simulink model "hopper_6dof_cascade_PID"  (R2025a)
settings: Solver=VariableStepAuto  StartTime=0.0  StopTime=36  RelTol=1e-3
undefined symbols (not defined in the file or in its folder): AVI, bp, ENGINE, IN, OUT, TANKS, tbl1, tbl2
libraries: slpidlib x13, dspindex x1, aerolibanim x1, SignalEditorBlockLib x1
(part 2 of 2)

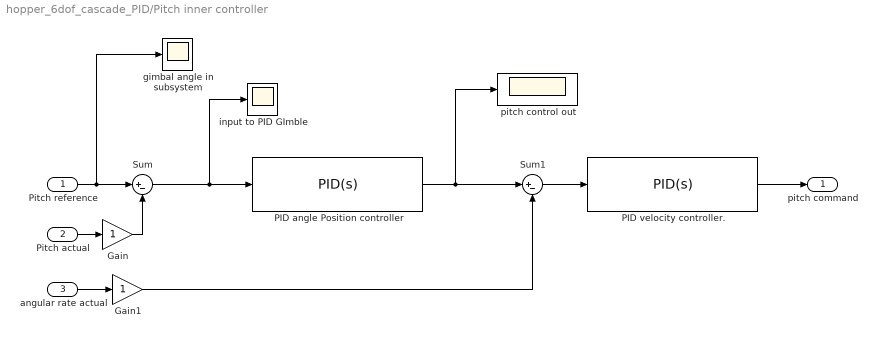
== system hopper_6dof_cascade_PID/Pitch inner controller ==
  Pitch reference : Inport
  Pitch actual : Inport  Port=2
  angular rate actual : Inport  Port=3
  Gain : Gain
  Gain1 : Gain
  PID angle Position controller : slpidlib/PID Controller  Controller=PID  Form=Parallel  TimeDomain=Continuous-time  UseExternalTs=off  SampleTime=.01  IntegratorMethod=Forward Euler  FilterMethod=Forward Euler  ControllerParametersSource=internal  P=2.71925952557616  I=0.432929489163779  UseKiTs=off  D=0.921646829283693  UseExternalDerivativeSource=off  N=202.456655722126  UseFilter=on  TunerSelectOption=Transfer Function Based (PID Tuner App)  InitialConditionSource=internal  InitialConditionForIntegrator=0  InitialConditionForFilter=0  DifferentiatorICPrevScaledInput=0  ExternalReset=none  TrackingMode=off  Kt=1  LimitOutput=off  SatLimitsSource=internal  UpperSaturationLimit=inf  LowerSaturationLimit=-inf  LinearizeAsGain=on  AntiWindupMode=none  Kb=1  LimitIntegrator=off  UpperIntegratorSaturationLimit=inf  LowerIntegratorSaturationLimit=-inf  POutMin=[]  POutMax=[]  IOutMin=[]  IOutMax=[]  DOutMin=[]  DOutMax=[]  NOutMin=[]  NOutMax=[]  SumOutMin=[]  SumOutMax=[]  SaturationOutMin=[]  SaturationOutMax=[]  PParamMin=[]  PParamMax=[]  IParamMin=[]  IParamMax=[]  DParamMin=[]  DParamMax=[]  NParamMin=[]  NParamMax=[]  KbParamMin=[]  KbParamMax=[]  KtParamMin=[]  KtParamMax=[]  KbOutMin=[]  KbOutMax=[]  KtOutMin=[]  KtOutMax=[]  IntegratorOutMin=[]  IntegratorOutMax=[]  FilterOutMin=[]  FilterOutMax=[]  SumI1OutMin=[]  SumI1OutMax=[]  SumI2OutMin=[]  SumI2OutMax=[]  SumI3OutMin=[]  SumI3OutMax=[]  SumI4OutMin=[]  SumI4OutMax=[]  SumDOutMin=[]  SumDOutMax=[]  DifferentiatorOutMin=[]  DifferentiatorOutMax=[]  FilterDiffOutCoefMin=[]  FilterDiffOutCoefMax=[]  ReciprocalOutMin=[]  ReciprocalOutMax=[]  SumDenOutMin=[]  SumDenOutMax=[]  SumNumOutMin=[]  SumNumOutMax=[]  DivideOutMin=[]  DivideOutMax=[]  UdiffTsProdOutMin=[]  UdiffTsProdOutMax=[]  NTsProdOutMin=[]  NTsProdOutMax=[]  UintegralTsProdOutMin=[]  UintegralTsProdOutMax=[]  UngainTsProdOutMin=[]  UngainTsProdOutMax=[]  ClampingZeroOutDataTypeStr=Inherit: Inherit via back propagation  ClampingZeroOutMin=[]  ClampingZeroOutMax=[]  FilterDenConstantOutDataTypeStr=Inherit: Inherit via back propagation  FilterDenConstantOutMin=[]  FilterDenConstantOutMax=[]  PCopyOutDataTypeStr=Inherit: Inherit via back propagation  PCopyOutMin=[]  PCopyOutMax=[]  NCopyOutDataTypeStr=Inherit: Inherit via back propagation  NCopyOutMin=[]  NCopyOutMax=[]  IntegratorContinuousStateAttributes=''  IntegratorStateMustResolveToSignalObject=off  IntegratorRTWStateStorageClass=Auto  FilterContinuousStateAttributes=''  FilterStateMustResolveToSignalObject=off  FilterRTWStateStorageClass=Auto  ParallelPVariant=InternalParameters  IdealPVariant=Disabled  IVariant=InternalParameters  DVariant=InternalParameters  IntegratorVariant=Continuous  SatVariant=Disabled  AWVariant=Passthrough  PCopyVariant=Disabled  TRVariant=Disabled  FdbkBlocksVariant=Forward  IdealPFdbkVariant=Disabled  SatFdbkVariant=Disabled  DerivativeFilterVariant=ContFilter  NVariant=InternalParameters  NCopyVariant=Disabled  FilterICVariant=InternalICsFilter  IntegratorICVariant=InternalICs  ExternalResetVariant=Disabled  TRSumVariant=Passthrough  SumFdbkVariant=Disabled  SumVariant=Sum_PID  TsampFilterVariant=InternalTs  TsampNgainVariant=Passthrough  TsampIntegralVariant=Disabled_SignalSpec  ExternalSaturationOutDataTypeStr=Inherit: Same as second input  DerivativeSourceVariant=ErrorSignal  PreIntVariant=InternalPreInt
  PID velocity controller. : slpidlib/PID Controller  Controller=PID  Form=Parallel  TimeDomain=Continuous-time  UseExternalTs=off  SampleTime=.01  IntegratorMethod=Forward Euler  FilterMethod=Forward Euler  ControllerParametersSource=internal  P=0.0125882721746036  I=0.00136230972396466  UseKiTs=off  D=0.023343460151588  UseExternalDerivativeSource=off  N=1.99025149076839  UseFilter=on  TunerSelectOption=Transfer Function Based (PID Tuner App)  InitialConditionSource=internal  InitialConditionForIntegrator=0  InitialConditionForFilter=0  DifferentiatorICPrevScaledInput=0  ExternalReset=none  TrackingMode=off  Kt=1  LimitOutput=off  SatLimitsSource=internal  UpperSaturationLimit=inf  LowerSaturationLimit=-inf  LinearizeAsGain=on  AntiWindupMode=none  Kb=1  LimitIntegrator=off  UpperIntegratorSaturationLimit=inf  LowerIntegratorSaturationLimit=-inf  POutMin=[]  POutMax=[]  IOutMin=[]  IOutMax=[]  DOutMin=[]  DOutMax=[]  NOutMin=[]  NOutMax=[]  SumOutMin=[]  SumOutMax=[]  SaturationOutMin=[]  SaturationOutMax=[]  PParamMin=[]  PParamMax=[]  IParamMin=[]  IParamMax=[]  DParamMin=[]  DParamMax=[]  NParamMin=[]  NParamMax=[]  KbParamMin=[]  KbParamMax=[]  KtParamMin=[]  KtParamMax=[]  KbOutMin=[]  KbOutMax=[]  KtOutMin=[]  KtOutMax=[]  IntegratorOutMin=[]  IntegratorOutMax=[]  FilterOutMin=[]  FilterOutMax=[]  SumI1OutMin=[]  SumI1OutMax=[]  SumI2OutMin=[]  SumI2OutMax=[]  SumI3OutMin=[]  SumI3OutMax=[]  SumI4OutMin=[]  SumI4OutMax=[]  SumDOutMin=[]  SumDOutMax=[]  DifferentiatorOutMin=[]  DifferentiatorOutMax=[]  FilterDiffOutCoefMin=[]  FilterDiffOutCoefMax=[]  ReciprocalOutMin=[]  ReciprocalOutMax=[]  SumDenOutMin=[]  SumDenOutMax=[]  SumNumOutMin=[]  SumNumOutMax=[]  DivideOutMin=[]  DivideOutMax=[]  UdiffTsProdOutMin=[]  UdiffTsProdOutMax=[]  NTsProdOutMin=[]  NTsProdOutMax=[]  UintegralTsProdOutMin=[]  UintegralTsProdOutMax=[]  UngainTsProdOutMin=[]  UngainTsProdOutMax=[]  ClampingZeroOutDataTypeStr=Inherit: Inherit via back propagation  ClampingZeroOutMin=[]  ClampingZeroOutMax=[]  FilterDenConstantOutDataTypeStr=Inherit: Inherit via back propagation  FilterDenConstantOutMin=[]  FilterDenConstantOutMax=[]  PCopyOutDataTypeStr=Inherit: Inherit via back propagation  PCopyOutMin=[]  PCopyOutMax=[]  NCopyOutDataTypeStr=Inherit: Inherit via back propagation  NCopyOutMin=[]  NCopyOutMax=[]  IntegratorContinuousStateAttributes=''  IntegratorStateMustResolveToSignalObject=off  IntegratorRTWStateStorageClass=Auto  FilterContinuousStateAttributes=''  FilterStateMustResolveToSignalObject=off  FilterRTWStateStorageClass=Auto  ParallelPVariant=InternalParameters  IdealPVariant=Disabled  IVariant=InternalParameters  DVariant=InternalParameters  IntegratorVariant=Continuous  SatVariant=Disabled  AWVariant=Passthrough  PCopyVariant=Disabled  TRVariant=Disabled  FdbkBlocksVariant=Forward  IdealPFdbkVariant=Disabled  SatFdbkVariant=Disabled  DerivativeFilterVariant=ContFilter  NVariant=InternalParameters  NCopyVariant=Disabled  FilterICVariant=InternalICsFilter  IntegratorICVariant=InternalICs  ExternalResetVariant=Disabled  TRSumVariant=Passthrough  SumFdbkVariant=Disabled  SumVariant=Sum_PID  TsampFilterVariant=InternalTs  TsampNgainVariant=Passthrough  TsampIntegralVariant=Disabled_SignalSpec  ExternalSaturationOutDataTypeStr=Inherit: Same as second input  DerivativeSourceVariant=ErrorSignal  PreIntVariant=InternalPreInt
  Sum : Sum  Inputs=|+-
  Sum1 : Sum  Inputs=|+-
  gimbal angle in subsystem : Scope
      settings: ActiveDisplayYMinimum=-0.050908038627042115  ActiveDisplayYMaximum=0.037591083917641  DataLoggingVariableName=ScopeData34
  input to PID GImble : Scope
      settings: ActiveDisplayYMinimum=-4.3031232761314806  ActiveDisplayYMaximum=2.5199807787902841  DataLoggingVariableName=ScopeData32
  pitch control out : Scope
      settings: ActiveDisplayYMinimum=6.4844722385980127E-5  ActiveDisplayYMaximum=0.015867649870164591  DataLoggingVariableName=ScopeData33
  pitch command : Outport
  wires:
  Pitch reference/1 -> gimbal angle in subsystem/1, Sum/1
  Pitch actual/1 -> Gain/1
  Gain/1 -> Sum/2
  Sum/1 -> input to PID GImble/1, PID angle Position controller/1
  PID angle Position controller/1 -> Sum1/1, pitch control out/1
  angular rate actual/1 -> Gain1/1
  Gain1/1 -> Sum1/2
  Sum1/1 -> PID velocity controller./1
  PID velocity controller./1 -> pitch command/1

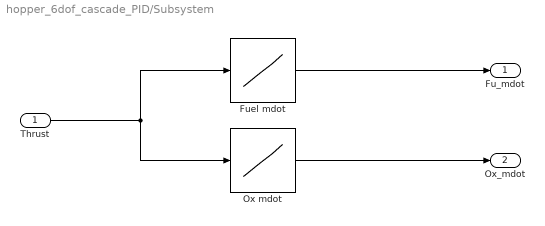
== system hopper_6dof_cascade_PID/Subsystem ==
  Thrust : Inport
  Fuel mdot : Lookup_n-D  NumberOfTableDimensions=1  BreakpointsForDimension1=bp  Table=tbl2  InternalRulePriority=Speed  RndMeth=Simplest
  Ox mdot : Lookup_n-D  NumberOfTableDimensions=1  BreakpointsForDimension1=bp  Table=tbl1  InternalRulePriority=Speed  RndMeth=Simplest
  Fu_mdot : Outport
  Ox_mdot : Outport  Port=2
  wires:
  Thrust/1 -> Ox mdot/1, Fuel mdot/1
  Fuel mdot/1 -> Fu_mdot/1
  Ox mdot/1 -> Ox_mdot/1

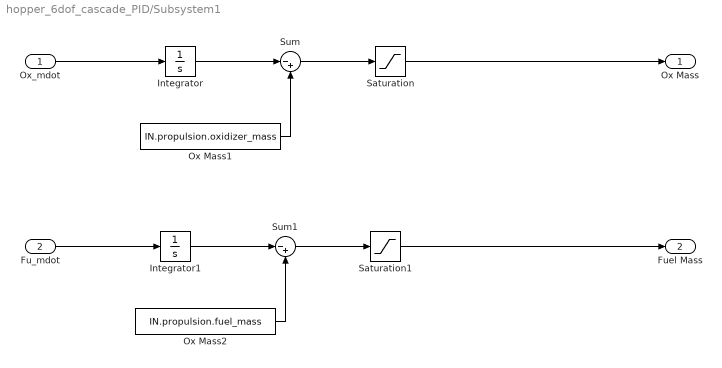
== system hopper_6dof_cascade_PID/Subsystem1 ==
  Ox_mdot : Inport
  Fu_mdot : Inport  Port=2
  Integrator : Integrator
  Integrator1 : Integrator
  Ox Mass1 : Constant  Value=IN.propulsion.oxidizer_mass
  Ox Mass2 : Constant  Value=IN.propulsion.fuel_mass
  Saturation : Saturate  UpperLimit=IN.propulsion.oxidizer_mass  LowerLimit=0
  Saturation1 : Saturate  UpperLimit=IN.propulsion.fuel_mass  LowerLimit=0
  Sum : Sum  Inputs=|-+
  Sum1 : Sum  Inputs=|-+
  Ox Mass : Outport
  Fuel Mass : Outport  Port=2
  wires:
  Ox_mdot/1 -> Integrator/1
  Integrator/1 -> Sum/1
  Ox Mass1/1 -> Sum/2
  Sum/1 -> Saturation/1
  Saturation/1 -> Ox Mass/1
  Sum1/1 -> Saturation1/1
  Saturation1/1 -> Fuel Mass/1
  Fu_mdot/1 -> Integrator1/1
  Ox Mass2/1 -> Sum1/2
  Integrator1/1 -> Sum1/1

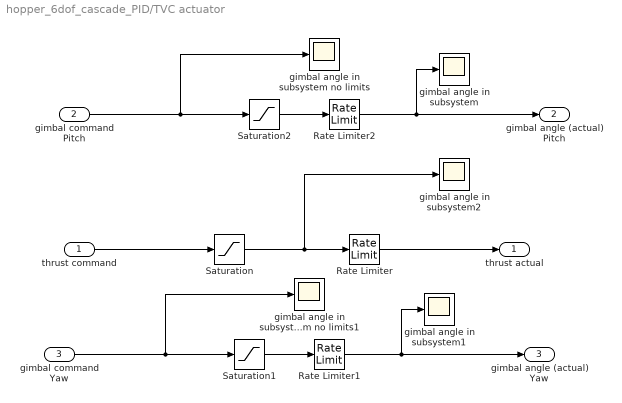
== system hopper_6dof_cascade_PID/TVC actuator ==
  thrust command : Inport
  gimbal command Pitch : Inport  Port=2
  gimbal command Yaw : Inport  Port=3
  Rate Limiter : RateLimiter  RisingSlewLimit=800  FallingSlewLimit=-800  SampleTimeMode=inherited
  Rate Limiter1 : RateLimiter  RisingSlewLimit=.2618  FallingSlewLimit=-.2618  SampleTimeMode=inherited
  Rate Limiter2 : RateLimiter  RisingSlewLimit=.2618  FallingSlewLimit=-.2618  SampleTimeMode=inherited
  Saturation : Saturate  UpperLimit=2400  LowerLimit=890
  Saturation1 : Saturate  UpperLimit=.2618  LowerLimit=-.2618
  Saturation2 : Saturate  UpperLimit=.2618  LowerLimit=-.2618
  gimbal angle in subsystem : Scope
      settings: ActiveDisplayYMinimum=-0.027763262466734467  ActiveDisplayYMaximum=0.0055911260638454568
  gimbal angle in subsystem no limits : Scope
      settings: ActiveDisplayYMinimum=-0.050908038627042115  ActiveDisplayYMaximum=0.037591083917641  DataLoggingVariableName=ScopeData28
  gimbal angle in subsystem no limits1 : Scope
      settings: ActiveDisplayYMinimum=-0.050908038627042115  ActiveDisplayYMaximum=0.037591083917641  DataLoggingVariableName=ScopeData31
  gimbal angle in subsystem1 : Scope
      settings: ActiveDisplayYMinimum=-0.027763262466734467  ActiveDisplayYMaximum=0.0055911260638454568  DataLoggingVariableName=ScopeData36
  gimbal angle in subsystem2 : Scope
      settings: ActiveDisplayYMinimum=-0.027763262466734467  ActiveDisplayYMaximum=0.0055911260638454568  DataLoggingVariableName=ScopeData35
  thrust actual : Outport
  gimbal angle (actual) Pitch : Outport  Port=2
  gimbal angle (actual) Yaw : Outport  Port=3
  wires:
  gimbal command Pitch/1 -> gimbal angle in subsystem no limits/1, Saturation2/1
  Saturation2/1 -> Rate Limiter2/1
  Rate Limiter2/1 -> gimbal angle (actual) Pitch/1, gimbal angle in subsystem/1
  Saturation/1 -> gimbal angle in subsystem2/1, Rate Limiter/1
  thrust command/1 -> Saturation/1
  Rate Limiter/1 -> thrust actual/1
  gimbal command Yaw/1 -> gimbal angle in subsystem no limits1/1, Saturation1/1
  Rate Limiter1/1 -> gimbal angle (actual) Yaw/1, gimbal angle in subsystem1/1
  Saturation1/1 -> Rate Limiter1/1

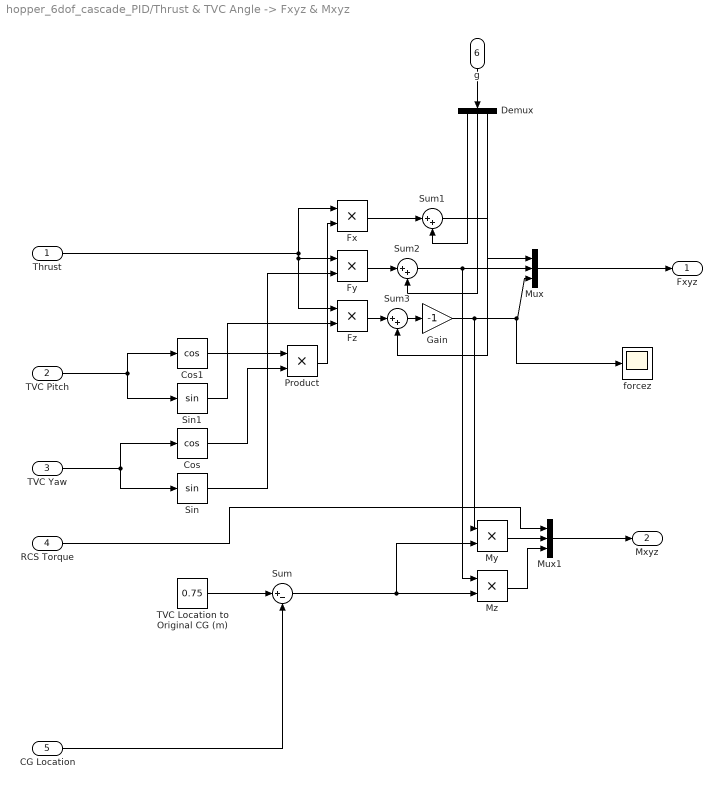
== system hopper_6dof_cascade_PID/Thrust & TVC Angle -> Fxyz & Mxyz ==
  "Thrust " : Inport
  TVC Pitch : Inport  Port=2
  TVC Yaw : Inport  Port=3
  RCS Torque : Inport  Port=4
  CG Location : Inport  Port=5
  g : Inport  Port=6
  Cos : Trigonometry  Operator=cos
  Cos1 : Trigonometry  Operator=cos
  Demux : Demux  Outputs=3
  Fx : Product
  Fy : Product
  Fz : Product
  Gain : Gain  Gain=-1
  Mux : Mux  Inputs=3
  Mux1 : Mux  Inputs=3
  My : Product
  Mz : Product
  Product : Product
  Sin : Trigonometry
  Sin1 : Trigonometry
  Sum : Sum  Inputs=|+-
  Sum1 : Sum  Inputs=|++
  Sum2 : Sum  Inputs=|++
  Sum3 : Sum  Inputs=|++
  TVC Location to Original CG (m) : Constant  Value=0.75
  forcez : Scope
      settings: ActiveDisplayYMinimum=-0.027763262466734467  ActiveDisplayYMaximum=0.0055911260638454568  DataLoggingVariableName=ScopeData37
  Fxyz : Outport
  Mxyz : Outport  Port=2
  wires:
  TVC Yaw/1 -> Sin/1, Cos/1
  TVC Pitch/1 -> Sin1/1, Cos1/1
  Cos1/1 -> Product/1
  Cos/1 -> Product/2
  Product/1 -> Fx/2
  "Thrust "/1 -> Fy/1, Fz/1, Fx/1
  Sin/1 -> Fy/2
  Sin1/1 -> Fz/2
  Mux/1 -> Fxyz/1
  TVC Location to Original CG (m)/1 -> Sum/1
  CG Location/1 -> Sum/2
  Sum/1 -> My/2, Mz/2
  RCS Torque/1 -> Mux1/1
  My/1 -> Mux1/2
  Mz/1 -> Mux1/3
  Mux1/1 -> Mxyz/1
  Gain/1 -> forcez/1, Mux/3, My/1
  Fx/1 -> Sum1/1
  Sum1/1 -> Mux/1
  g/1 -> Demux/1
  Demux/1 -> Sum1/2
  Fy/1 -> Sum2/1
  Sum2/1 -> Mz/1, Mux/2
  Fz/1 -> Sum3/1
  Sum3/1 -> Gain/1
  Demux/2 -> Sum2/2
  Demux/3 -> Sum3/2

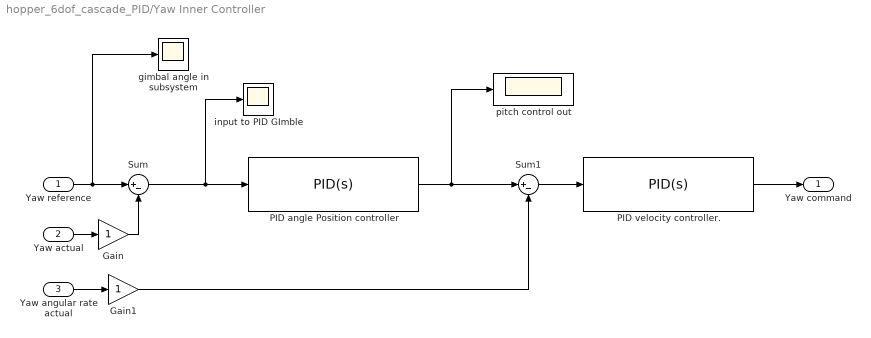
== system hopper_6dof_cascade_PID/Yaw Inner Controller ==
  Yaw reference : Inport
  Yaw actual : Inport  Port=2
  Yaw angular rate actual : Inport  Port=3
  Gain : Gain
  Gain1 : Gain
  PID angle Position controller : slpidlib/PID Controller  Controller=PID  Form=Parallel  TimeDomain=Continuous-time  UseExternalTs=off  SampleTime=.01  IntegratorMethod=Forward Euler  FilterMethod=Forward Euler  ControllerParametersSource=internal  P=2.71925952557616  I=0.432929489163779  UseKiTs=off  D=0.921646829283693  UseExternalDerivativeSource=off  N=202.456655722126  UseFilter=on  TunerSelectOption=Transfer Function Based (PID Tuner App)  InitialConditionSource=internal  InitialConditionForIntegrator=0  InitialConditionForFilter=0  DifferentiatorICPrevScaledInput=0  ExternalReset=none  TrackingMode=off  Kt=1  LimitOutput=off  SatLimitsSource=internal  UpperSaturationLimit=inf  LowerSaturationLimit=-inf  LinearizeAsGain=on  AntiWindupMode=none  Kb=1  LimitIntegrator=off  UpperIntegratorSaturationLimit=inf  LowerIntegratorSaturationLimit=-inf  POutMin=[]  POutMax=[]  IOutMin=[]  IOutMax=[]  DOutMin=[]  DOutMax=[]  NOutMin=[]  NOutMax=[]  SumOutMin=[]  SumOutMax=[]  SaturationOutMin=[]  SaturationOutMax=[]  PParamMin=[]  PParamMax=[]  IParamMin=[]  IParamMax=[]  DParamMin=[]  DParamMax=[]  NParamMin=[]  NParamMax=[]  KbParamMin=[]  KbParamMax=[]  KtParamMin=[]  KtParamMax=[]  KbOutMin=[]  KbOutMax=[]  KtOutMin=[]  KtOutMax=[]  IntegratorOutMin=[]  IntegratorOutMax=[]  FilterOutMin=[]  FilterOutMax=[]  SumI1OutMin=[]  SumI1OutMax=[]  SumI2OutMin=[]  SumI2OutMax=[]  SumI3OutMin=[]  SumI3OutMax=[]  SumI4OutMin=[]  SumI4OutMax=[]  SumDOutMin=[]  SumDOutMax=[]  DifferentiatorOutMin=[]  DifferentiatorOutMax=[]  FilterDiffOutCoefMin=[]  FilterDiffOutCoefMax=[]  ReciprocalOutMin=[]  ReciprocalOutMax=[]  SumDenOutMin=[]  SumDenOutMax=[]  SumNumOutMin=[]  SumNumOutMax=[]  DivideOutMin=[]  DivideOutMax=[]  UdiffTsProdOutMin=[]  UdiffTsProdOutMax=[]  NTsProdOutMin=[]  NTsProdOutMax=[]  UintegralTsProdOutMin=[]  UintegralTsProdOutMax=[]  UngainTsProdOutMin=[]  UngainTsProdOutMax=[]  ClampingZeroOutDataTypeStr=Inherit: Inherit via back propagation  ClampingZeroOutMin=[]  ClampingZeroOutMax=[]  FilterDenConstantOutDataTypeStr=Inherit: Inherit via back propagation  FilterDenConstantOutMin=[]  FilterDenConstantOutMax=[]  PCopyOutDataTypeStr=Inherit: Inherit via back propagation  PCopyOutMin=[]  PCopyOutMax=[]  NCopyOutDataTypeStr=Inherit: Inherit via back propagation  NCopyOutMin=[]  NCopyOutMax=[]  IntegratorContinuousStateAttributes=''  IntegratorStateMustResolveToSignalObject=off  IntegratorRTWStateStorageClass=Auto  FilterContinuousStateAttributes=''  FilterStateMustResolveToSignalObject=off  FilterRTWStateStorageClass=Auto  ParallelPVariant=InternalParameters  IdealPVariant=Disabled  IVariant=InternalParameters  DVariant=InternalParameters  IntegratorVariant=Continuous  SatVariant=Disabled  AWVariant=Passthrough  PCopyVariant=Disabled  TRVariant=Disabled  FdbkBlocksVariant=Forward  IdealPFdbkVariant=Disabled  SatFdbkVariant=Disabled  DerivativeFilterVariant=ContFilter  NVariant=InternalParameters  NCopyVariant=Disabled  FilterICVariant=InternalICsFilter  IntegratorICVariant=InternalICs  ExternalResetVariant=Disabled  TRSumVariant=Passthrough  SumFdbkVariant=Disabled  SumVariant=Sum_PID  TsampFilterVariant=InternalTs  TsampNgainVariant=Passthrough  TsampIntegralVariant=Disabled_SignalSpec  ExternalSaturationOutDataTypeStr=Inherit: Same as second input  DerivativeSourceVariant=ErrorSignal  PreIntVariant=InternalPreInt
  PID velocity controller. : slpidlib/PID Controller  Controller=PID  Form=Parallel  TimeDomain=Continuous-time  UseExternalTs=off  SampleTime=.01  IntegratorMethod=Forward Euler  FilterMethod=Forward Euler  ControllerParametersSource=internal  P=0.0125882721746036  I=0.00136230972396466  UseKiTs=off  D=0.023343460151588  UseExternalDerivativeSource=off  N=1.99025149076839  UseFilter=on  TunerSelectOption=Transfer Function Based (PID Tuner App)  InitialConditionSource=internal  InitialConditionForIntegrator=0  InitialConditionForFilter=0  DifferentiatorICPrevScaledInput=0  ExternalReset=none  TrackingMode=off  Kt=1  LimitOutput=off  SatLimitsSource=internal  UpperSaturationLimit=inf  LowerSaturationLimit=-inf  LinearizeAsGain=on  AntiWindupMode=none  Kb=1  LimitIntegrator=off  UpperIntegratorSaturationLimit=inf  LowerIntegratorSaturationLimit=-inf  POutMin=[]  POutMax=[]  IOutMin=[]  IOutMax=[]  DOutMin=[]  DOutMax=[]  NOutMin=[]  NOutMax=[]  SumOutMin=[]  SumOutMax=[]  SaturationOutMin=[]  SaturationOutMax=[]  PParamMin=[]  PParamMax=[]  IParamMin=[]  IParamMax=[]  DParamMin=[]  DParamMax=[]  NParamMin=[]  NParamMax=[]  KbParamMin=[]  KbParamMax=[]  KtParamMin=[]  KtParamMax=[]  KbOutMin=[]  KbOutMax=[]  KtOutMin=[]  KtOutMax=[]  IntegratorOutMin=[]  IntegratorOutMax=[]  FilterOutMin=[]  FilterOutMax=[]  SumI1OutMin=[]  SumI1OutMax=[]  SumI2OutMin=[]  SumI2OutMax=[]  SumI3OutMin=[]  SumI3OutMax=[]  SumI4OutMin=[]  SumI4OutMax=[]  SumDOutMin=[]  SumDOutMax=[]  DifferentiatorOutMin=[]  DifferentiatorOutMax=[]  FilterDiffOutCoefMin=[]  FilterDiffOutCoefMax=[]  ReciprocalOutMin=[]  ReciprocalOutMax=[]  SumDenOutMin=[]  SumDenOutMax=[]  SumNumOutMin=[]  SumNumOutMax=[]  DivideOutMin=[]  DivideOutMax=[]  UdiffTsProdOutMin=[]  UdiffTsProdOutMax=[]  NTsProdOutMin=[]  NTsProdOutMax=[]  UintegralTsProdOutMin=[]  UintegralTsProdOutMax=[]  UngainTsProdOutMin=[]  UngainTsProdOutMax=[]  ClampingZeroOutDataTypeStr=Inherit: Inherit via back propagation  ClampingZeroOutMin=[]  ClampingZeroOutMax=[]  FilterDenConstantOutDataTypeStr=Inherit: Inherit via back propagation  FilterDenConstantOutMin=[]  FilterDenConstantOutMax=[]  PCopyOutDataTypeStr=Inherit: Inherit via back propagation  PCopyOutMin=[]  PCopyOutMax=[]  NCopyOutDataTypeStr=Inherit: Inherit via back propagation  NCopyOutMin=[]  NCopyOutMax=[]  IntegratorContinuousStateAttributes=''  IntegratorStateMustResolveToSignalObject=off  IntegratorRTWStateStorageClass=Auto  FilterContinuousStateAttributes=''  FilterStateMustResolveToSignalObject=off  FilterRTWStateStorageClass=Auto  ParallelPVariant=InternalParameters  IdealPVariant=Disabled  IVariant=InternalParameters  DVariant=InternalParameters  IntegratorVariant=Continuous  SatVariant=Disabled  AWVariant=Passthrough  PCopyVariant=Disabled  TRVariant=Disabled  FdbkBlocksVariant=Forward  IdealPFdbkVariant=Disabled  SatFdbkVariant=Disabled  DerivativeFilterVariant=ContFilter  NVariant=InternalParameters  NCopyVariant=Disabled  FilterICVariant=InternalICsFilter  IntegratorICVariant=InternalICs  ExternalResetVariant=Disabled  TRSumVariant=Passthrough  SumFdbkVariant=Disabled  SumVariant=Sum_PID  TsampFilterVariant=InternalTs  TsampNgainVariant=Passthrough  TsampIntegralVariant=Disabled_SignalSpec  ExternalSaturationOutDataTypeStr=Inherit: Same as second input  DerivativeSourceVariant=ErrorSignal  PreIntVariant=InternalPreInt
  Sum : Sum  Inputs=|+-
  Sum1 : Sum  Inputs=|+-
  gimbal angle in subsystem : Scope
      settings: ActiveDisplayYMinimum=-0.050908038627042115  ActiveDisplayYMaximum=0.037591083917641  DataLoggingVariableName=ScopeData34
  input to PID GImble : Scope
      settings: ActiveDisplayYMinimum=-4.3031232761314806  ActiveDisplayYMaximum=2.5199807787902841  DataLoggingVariableName=ScopeData32
  pitch control out : Scope
      settings: ActiveDisplayYMinimum=6.4844722385980127E-5  ActiveDisplayYMaximum=0.015867649870164591  DataLoggingVariableName=ScopeData33
  Yaw command : Outport
  wires:
  Yaw reference/1 -> gimbal angle in subsystem/1, Sum/1
  Yaw actual/1 -> Gain/1
  Gain/1 -> Sum/2
  Sum/1 -> input to PID GImble/1, PID angle Position controller/1
  PID angle Position controller/1 -> Sum1/1, pitch control out/1
  Yaw angular rate actual/1 -> Gain1/1
  Gain1/1 -> Sum1/2
  Sum1/1 -> PID velocity controller./1
  PID velocity controller./1 -> Yaw command/1

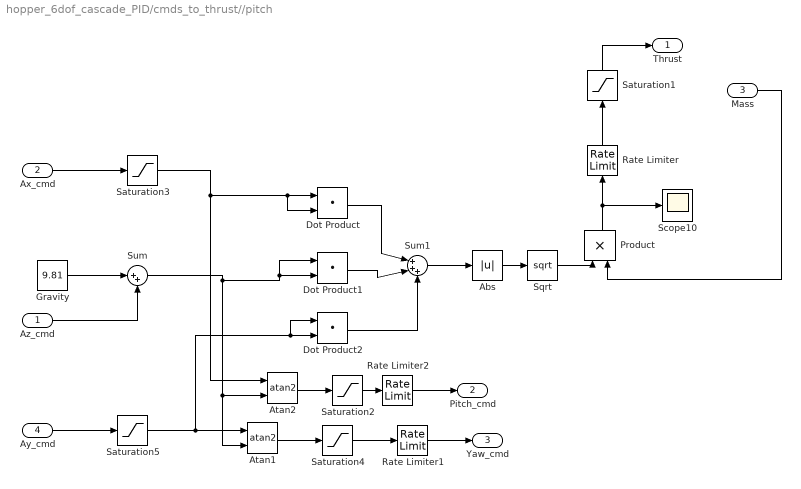
== system hopper_6dof_cascade_PID/cmds_to_thrust//pitch ==
  Az_cmd : Inport
  Ax_cmd : Inport  Port=2
  Mass : Inport  Port=3
  Ay_cmd : Inport  Port=4
  Abs : Abs  SaturateOnIntegerOverflow=off
  Atan1 : Trigonometry  Operator=atan2
  Atan2 : Trigonometry  Operator=atan2
  Dot Product : DotProduct  OutDataTypeStr=Inherit: Inherit via internal rule
  Dot Product1 : DotProduct  OutDataTypeStr=Inherit: Inherit via internal rule
  Dot Product2 : DotProduct  OutDataTypeStr=Inherit: Inherit via internal rule
  Gravity : Constant  Value=9.81
  Product : Product
  Rate Limiter : RateLimiter  RisingSlewLimit=800  FallingSlewLimit=-800  SampleTimeMode=inherited
  Rate Limiter1 : RateLimiter  RisingSlewLimit=.2618  FallingSlewLimit=-.2618  SampleTimeMode=inherited
  Rate Limiter2 : RateLimiter  RisingSlewLimit=.2618  FallingSlewLimit=-.2618  SampleTimeMode=inherited
  Saturation1 : Saturate  UpperLimit=2400  LowerLimit=890  ZeroCross=off
  Saturation2 : Saturate  UpperLimit=.1  LowerLimit=-.1
  Saturation3 : Saturate  UpperLimit=.8  LowerLimit=-.8
  Saturation4 : Saturate  UpperLimit=.1  LowerLimit=-.1
  Saturation5 : Saturate  UpperLimit=.8  LowerLimit=-.8
  Scope10 : Scope
      settings: ActiveDisplayYMinimum=-1  ActiveDisplayYMaximum=1  DataLoggingVariableName=ScopeData18
  Sqrt : Sqrt
  Sum : Sum  Inputs=|++
  Sum1 : Sum  Inputs=|+++
  Thrust : Outport
  Pitch_cmd : Outport  Port=2
  Yaw_cmd : Outport  Port=3
  wires:
  Dot Product/1 -> Sum1/1
  Gravity/1 -> Sum/1
  Atan2/1 -> Saturation2/1
  Saturation2/1 -> Rate Limiter2/1
  Product/1 -> Scope10/1, Rate Limiter/1
  Rate Limiter2/1 -> Pitch_cmd/1
  Dot Product1/1 -> Sum1/2
  Sum/1 -> Dot Product1/1, Dot Product1/2, Atan2/2, Atan1/2
  Sum1/1 -> Abs/1
  Ax_cmd/1 -> Saturation3/1
  Saturation3/1 -> Dot Product/2, Dot Product/1, Atan2/1
  Rate Limiter/1 -> Saturation1/1
  Sqrt/1 -> Product/1
  Abs/1 -> Sqrt/1
  Saturation1/1 -> Thrust/1
  Mass/1 -> Product/2
  Az_cmd/1 -> Sum/2
  Ay_cmd/1 -> Saturation5/1
  Atan1/1 -> Saturation4/1
  Saturation4/1 -> Rate Limiter1/1
  Rate Limiter1/1 -> Yaw_cmd/1
  Dot Product2/1 -> Sum1/3
  Saturation5/1 -> Atan1/1, Dot Product2/1, Dot Product2/2

== matlab function hopper_6dof_cascade_PID/CG // MOI Script v2/MATLAB Function ==
  data: ox_mass input; cg output; fu_mass input; engine_mass input; engine_cg input; ox_tank_mass input; ox_tank_cg input; ox_tank_wall_thick input; fu_tank_mass input; fu_tank_cg input; fu_tank_wall_thick input; structures_mass input; structures_cg input; avi_mass input; avi_cg input; fluids_mass input; fluids_cg input; payload_mass input; payload_cg input; ox_tank_h input; fu_tank_h input; tank_r input; it_h input; MoI output; copv_mass input; copv_r input; copv_t input; copv_h input; copv_zcg input; copv_ycg input
function [cg, MoI] = cg_sim(ox_mass, fu_mass, engine_mass, engine_cg, ox_tank_mass, ox_tank_cg, ox_tank_wall_thick, fu_tank_mass, fu_tank_cg, fu_tank_wall_thick, structures_mass, structures_cg, avi_mass, avi_cg, fluids_mass, fluids_cg, payload_mass, payload_cg, ox_tank_h, fu_tank_h, tank_r, it_h, copv_mass, copv_r, copv_t, copv_h, copv_zcg, copv_ycg)
%CG_SIM Calculates the Center of Gravity and Moment of Inertia Matrix
%   Inputs are masses (kg), CG positions (m), and dimensions (m).

    %% 1. Constants and Unit Conversions
    ox_density = 1141;   % kg/m^3
    fu_density = 800;    % kg/m^3
    al_density = 2700;   % kg/m^3 (Density of Al6061)
    
    % Engine dimensions: 4 inch radius, 1 ft length
    eng_r = 4 * 0.0254;  % inches to meters
    eng_h = 1 * 0.3048;  % ft to meters

    %% 2. End Cap Geometry & Mass (NEW)
    % Modeled as solid cylinders attached to the ends of the tank shells.
    % Height of cap = wall thickness of the respective tank.
    
    % --- Oxidizer Tank Caps ---
    h_ox_cap = ox_tank_wall_thick;
    vol_ox_cap = pi * tank_r^2 * h_ox_cap;
    m_ox_cap   = al_density * vol_ox_cap; % Mass of ONE cap
    
    % Positions (Top and Bottom of the hollow shell)
    % Z = Tank_CG +/- (Tank_H/2 + Cap_H/2)
    z_ox_cap_bot = ox_tank_cg - (ox_tank_h / 2) - (h_ox_cap / 2);
    z_ox_cap_top = ox_tank_cg + (ox_tank_h / 2) + (h_ox_cap / 2);

    % --- Fuel Tank Caps ---
    h_fu_cap = fu_tank_wall_thick;
    vol_fu_cap = pi * tank_r^2 * h_fu_cap;
    m_fu_cap   = al_density * vol_fu_cap; % Mass of ONE cap
    
    % Positions
    z_fu_cap_bot = fu_tank_cg - (fu_tank_h / 2) - (h_fu_cap / 2);
    z_fu_cap_top = fu_tank_cg + (fu_tank_h / 2) + (h_fu_cap / 2);

    %% 3. Fluid Geometry Calculations
    % Fuel Fluid
    if fu_mass > 0
        h_fu_fluid = (fu_mass / fu_density) / (pi * tank_r^2);
        % Fluid sits at the bottom of the tank shell
        z_fu_fluid = (fu_tank_cg - fu_tank_h/2) + (h_fu_fluid / 2);
    else
        h_fu_fluid = 0; z_fu_fluid = 0;
    end

    % Oxidizer Fluid
    if ox_mass > 0
        h_ox_fluid = (ox_mass / ox_density) / (pi * tank_r^2);
        z_ox_fluid = (ox_tank_cg - ox_tank_h/2) + (h_ox_fluid / 2);
    else
        h_ox_fluid = 0; z_ox_fluid = 0;
    end

    %% 4. Calculate System Center of Gravity (CG)
    % Sum of Moments = sum(mass * position)
    moment_sum = ...
        engine_mass * engine_cg + ...
        fu_tank_mass * fu_tank_cg + ...
        ox_tank_mass * ox_tank_cg + ...
        copv_mass * copv_zcg + ...
        structures_mass * structures_cg + ...
        avi_mass * avi_cg + ...
        fluids_mass * fluids_cg + ...
        payload_mass * payload_cg + ...
        fu_mass * z_fu_fluid + ...
        ox_mass * z_ox_fluid + ...
        m_ox_cap * z_ox_cap_bot + ... 
        m_ox_cap * z_ox_cap_top + ...  
        m_fu_cap * z_fu_cap_bot + ...  
        m_fu_cap * z_fu_cap_top;      

    total_mass = engine_mass + fu_tank_mass + ox_tank_mass +  copv_mass +...
                 structures_mass + avi_mass + fu_mass + ox_mass + fluids_mass + payload_mass +...
                 2 * m_ox_cap + 2 * m_fu_cap;

    if total_mass > 0
        cg = moment_sum / total_mass; % return 1
    else
        cg = 0;
    end

    %% 5. Calculate Moments of Inertia (MoI)
    % Anonymous functions for inertia - shout out gemini for this one
    calc_solid_Izz = @(m, r) 0.5 * m * r^2;
    calc_solid_Ixx = @(m, r, h) (1/12) * m * (3*r^2 + h^2);
    calc_hollow_Izz = @(m, ro, ri) 0.5 * m * (ro^2 + ri^2);
    calc_hollow_Ixx = @(m, ro, ri, h) (1/12) * m * (3*(ro^2 + ri^2) + h^2);

    % --- A. Engine ---
    Izz_eng = calc_solid_Izz(engine_mass, eng_r);
    Ixx_eng = calc_solid_Ixx(engine_mass, eng_r, eng_h) + engine_mass * (engine_cg - cg)^2;

    % --- B. Fuel Tank (Hollow Shell) ---
    r_in_fu = tank_r - fu_tank_wall_thick;
    Izz_fut = calc_hollow_Izz(fu_tank_mass, tank_r, r_in_fu);
    Ixx_fut = calc_hollow_Ixx(fu_tank_mass, tank_r, r_in_fu, fu_tank_h) + fu_tank_mass * (fu_tank_cg - cg)^2;

    % --- C. Oxidizer Tank (Hollow Shell) ---
    r_in_ox = tank_r - ox_tank_wall_thick;
    Izz_oxt = calc_hollow_Izz(ox_tank_mass, tank_r, r_in_ox);
    Ixx_oxt = calc_hollow_Ixx(ox_tank_mass, tank_r, r_in_ox, ox_tank_h) + ox_tank_mass * (ox_tank_cg - cg)^2;

    % --- D. COPV (Hollow Shell) ---
    r_in_copv = copv_r - copv_t;
    Izz_copvt = calc_hollow_Izz(copv_mass, copv_r, r_in_copv);
    Ixx_copvt = calc_hollow_Ixx(copv_mass,copv_r, r_in_copv, copv_h) + copv_mass * (copv_zcg - cg)^2

    % --- E. Structures --- just asssume cylinder in it
    Izz_str = calc_solid_Izz(structures_mass, tank_r);
    Ixx_str = calc_solid_Ixx(structures_mass, tank_r, it_h) + structures_mass * (structures_cg - cg)^2;

    % --- F. Avionics --- just asssume cylinder in it
    Izz_avi = calc_solid_Izz(avi_mass, tank_r);
    Ixx_avi = calc_solid_Ixx(avi_mass, tank_r, it_h) + avi_mass * (avi_cg - cg)^2;

    % --- G. Fluids System --- just asssume cylinder in it
    Izz_fluids = calc_solid_Izz(fluids_mass, tank_r);
    Ixx_fluids = calc_solid_Ixx(fluids_mass, tank_r, it_h) + fluids_mass * (fluids_cg - cg)^2;

    % --- H. Payload --- just asssume cylinder in it
    Izz_payload = calc_solid_Izz(payload_mass, tank_r);
    Ixx_payload = calc_solid_Ixx(payload_mass, tank_r, it_h) + payload_mass * (payload_cg - cg)^2;

    % --- I. Fluids ---
    if fu_mass > 0
        Izz_fuf = calc_solid_Izz(fu_mass, tank_r);
        Ixx_fuf = calc_solid_Ixx(fu_mass, tank_r, h_fu_fluid) + fu_mass * (z_fu_fluid - cg)^2;
    else
        Izz_fuf = 0; Ixx_fuf = 0;
    end

    if ox_mass > 0
        Izz_oxf = calc_solid_Izz(ox_mass, tank_r);
        Ixx_oxf = calc_solid_Ixx(ox_mass, tank_r, h_ox_fluid) + ox_mass * (z_ox_fluid - cg)^2;
    else
        Izz_oxf = 0; Ixx_oxf = 0;
    end

    % --- G. End Caps ---
    % 1. Ox Caps (Solid Cylinders)
    % Izz is same for both
    Izz_ox_cap = calc_solid_Izz(m_ox_cap, tank_r);
    Ixx_ox_cap_local = calc_solid_Ixx(m_ox_cap, tank_r, h_ox_cap);
    
    Ixx_ox_caps_total = ...
        (Ixx_ox_cap_local + m_ox_cap * (z_ox_cap_bot - cg)^2) + ... % Bottom Cap
        (Ixx_ox_cap_local + m_ox_cap * (z_ox_cap_top - cg)^2);      % Top Cap

    % 2. Fuel Caps (Solid Cylinders)
    Izz_fu_cap = calc_solid_Izz(m_fu_cap, tank_r);
    Ixx_fu_cap_local = calc_solid_Ixx(m_fu_cap, tank_r, h_fu_cap);
    
    Ixx_fu_caps_total = ...
        (Ixx_fu_cap_local + m_fu_cap * (z_fu_cap_bot - cg)^2) + ... % Bottom Cap
        (Ixx_fu_cap_local + m_fu_cap * (z_fu_cap_top - cg)^2);      % Top Cap

    %% 6. Summation
    Izz_total = Izz_eng + Izz_fut + Izz_oxt + Izz_str + Izz_avi + Izz_fluids + Izz_payload + Izz_copvt + ...
                Izz_fuf + Izz_oxf + ...
                2*Izz_ox_cap + 2*Izz_fu_cap;
                
    Ixx_total = Ixx_eng + Ixx_fut + Ixx_oxt + Ixx_str + Ixx_avi + Ixx_fluids + Ixx_payload + Ixx_copvt +...
                Ixx_fuf + Ixx_oxf + ...
                Ixx_ox_caps_total + Ixx_fu_caps_total;
    
    Iyy_total = Ixx_total + ...
        2 * Ixx_copvt * (copv_ycg)^2;
                

    MoI = [Izz_total, 0, 0; 
           0, Iyy_total, 0; 
           0, 0, Ixx_total]; % return 2
end
